simulink model "tp1_1"  (R2023b)
settings: Solver=VariableStepAuto  StartTime=0.0  StopTime=50  RelTol=1e-3
settings Model: Creator=rusha  LastModifiedBy=rusha

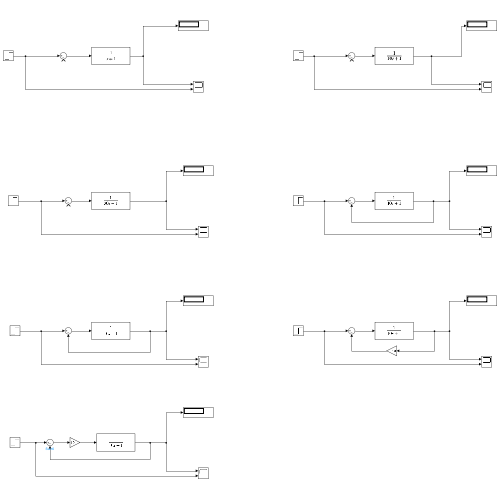
[thumbnail: Simulink's stored preview of the top-level diagram]
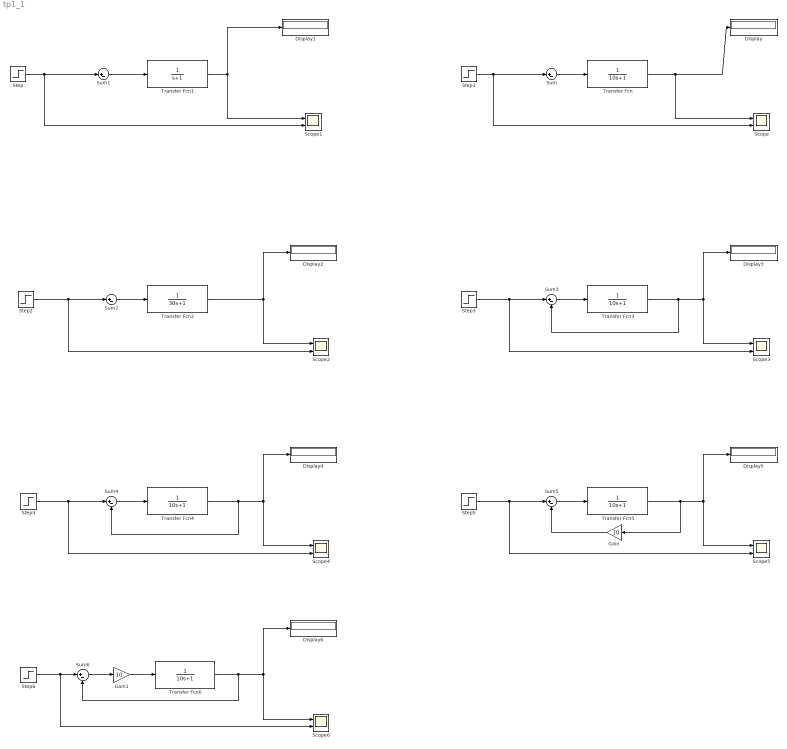
== system tp1_1 ==
  Display{,1..6} (7 alike) : Display
  Gain : Gain  Gain=10
  Gain1 : Gain  Gain=10
  Scope{,1..6} (7 alike) : Scope  NumInputPorts=2
  Step{,1..6} (7 alike) : Step  SampleTime=0
  Sum{,1..6} (7 alike) : Sum  Inputs=|+-
  Transfer Fcn{,3..6} (5 alike) : TransferFcn  Denominator=[10 1]
  Transfer Fcn1 : TransferFcn  Denominator=[1 1]
  Transfer Fcn2 : TransferFcn  Denominator=[30 1]
  wires:
  Step1/1 -> Scope/2, Sum/1
  Transfer Fcn/1 -> Display/1, Scope/1
  Sum/1 -> Transfer Fcn/1
  Transfer Fcn1/1 -> Display1/1, Scope1/1
  Step/1 -> Scope1/2, Sum1/1
  Sum1/1 -> Transfer Fcn1/1
  Sum2/1 -> Transfer Fcn2/1
  Transfer Fcn2/1 -> Display2/1, Scope2/1
  Step2/1 -> Scope2/2, Sum2/1
  Sum3/1 -> Transfer Fcn3/1
  Transfer Fcn3/1 -> Sum3/2, Display3/1, Scope3/1
  Step3/1 -> Scope3/2, Sum3/1
  Step4/1 -> Scope4/2, Sum4/1
  Sum4/1 -> Transfer Fcn4/1
  Transfer Fcn4/1 -> Sum4/2, Display4/1, Scope4/1
  Step5/1 -> Scope5/2, Sum5/1
  Sum5/1 -> Transfer Fcn5/1
  Transfer Fcn5/1 -> Gain/1, Display5/1, Scope5/1
  Gain/1 -> Sum5/2
  Step6/1 -> Scope6/2, Sum6/1
  Transfer Fcn6/1 -> Sum6/2, Display6/1, Scope6/1
  Sum6/1 -> Gain1/1
  Gain1/1 -> Transfer Fcn6/1
